simulink library "tramontina_database_moboticlib"  (R2024a)
settings: Solver=VariableStepAuto  StartTime=0.0  StopTime=10.0  RelTol=1e-3
libraries: canmsglib x4, simulink x1
settings Model: Creator=matlab.cut  LastModifiedBy=matlab.cut

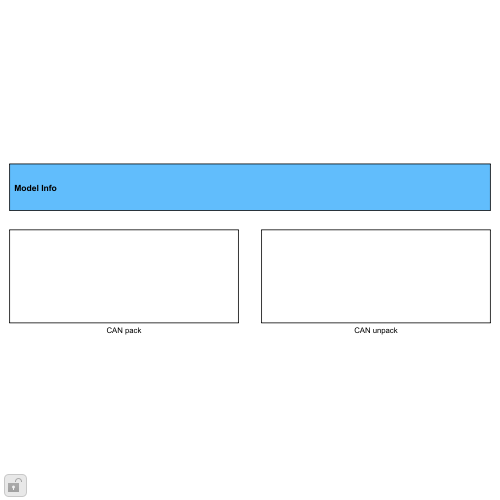
[thumbnail: Simulink's stored preview of the top-level diagram]
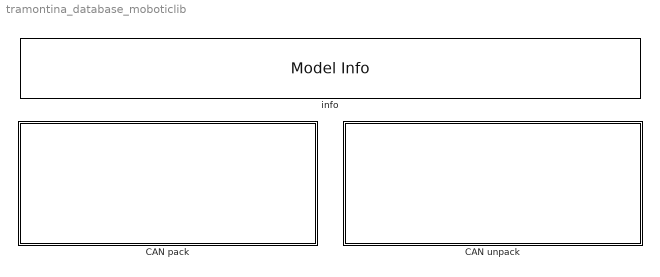
== system tramontina_database_moboticlib ==
  CAN pack : Subsystem
  CAN unpack : Subsystem
  info : simulink/Model-Wide Utilities/Model Info  Frame=on  DisplayStringWithTags=SPEEDGOAT CAN Database Library for: tramontina_database_mobotic  HorizontalTextAlignment=Left  LeftAlignmentValue=0.01

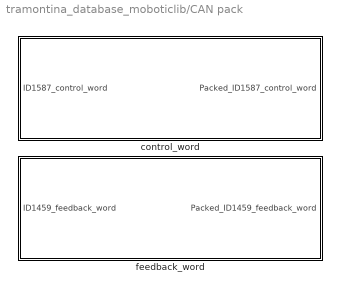
== system tramontina_database_moboticlib/CAN pack ==
  control_word : Subsystem
  feedback_word : Subsystem

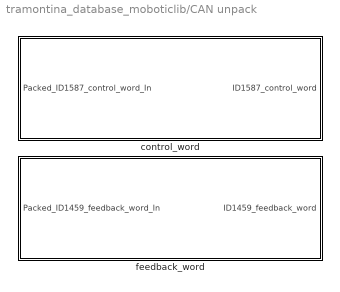
== system tramontina_database_moboticlib/CAN unpack ==
  control_word : Subsystem
  feedback_word : Subsystem

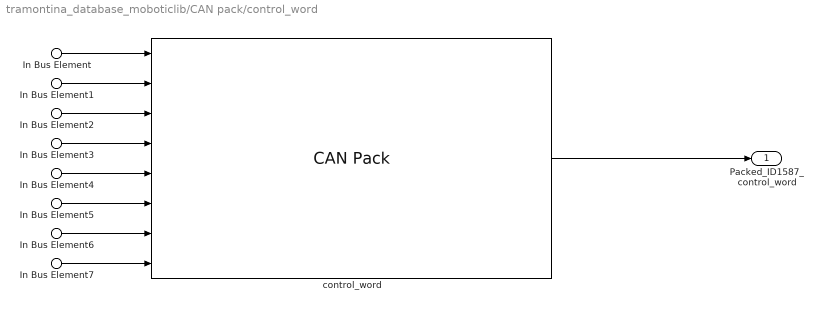
== system tramontina_database_moboticlib/CAN pack/control_word ==
  In Bus Element : Inport  PortName=ID1587_control_word  Element=byte0
  In Bus Element1 : Inport  PortName=ID1587_control_word  Element=byte1
  In Bus Element2 : Inport  PortName=ID1587_control_word  Element=byte2
  In Bus Element3 : Inport  PortName=ID1587_control_word  Element=byte3
  In Bus Element4 : Inport  PortName=ID1587_control_word  Element=byte4
  In Bus Element5 : Inport  PortName=ID1587_control_word  Element=byte5
  In Bus Element6 : Inport  PortName=ID1587_control_word  Element=byte6
  In Bus Element7 : Inport  PortName=ID1587_control_word  Element=byte7
  control_word : canmsglib/CAN Pack  CANdbFile=C:\Users\matlab.cut\Desktop\matlab\AMR_tramontina\Data\DBCFiles\tramontina_database_mobotic.dbc  MsgList=control_word  MsgName=control_word  MsgIDType=Standard (11-bit identifier)  MsgIdentifier=1587  MsgLength=8  Remote=off  ApplyMinMax=off  BusOutput=on  SignalInfo={'byte0','0','8','LE','unsigned','Standard','0','1','0','-Inf','Inf';'byte1','8','8','LE','unsigned','Standard','0','1','0','-Inf','Inf';'byte2','16','8','LE','unsigned','Standard','0','1','0','-Inf','Inf';'byte3','24','8','LE','unsigned','Standard','0','1','0','-Inf','Inf';'byte4','32','8','LE','unsigned','Standard','0','1','0','-Inf','Inf';'byte5','40','8','LE','unsigned','Standard','0','1','0','-Inf','Inf';'byte6','48','8','LE','unsigned','Standard','0','1','0','-Inf','Inf';'byte7','56','8','LE','unsigned','Standard','0','1','0','-Inf','Inf'}
      settings: DataFormat=manually specified signals
  Packed_ID1587_control_word : Outport
  wires:
  control_word/1 -> Packed_ID1587_control_word/1
  In Bus Element/1 -> control_word/1
  In Bus Element1/1 -> control_word/2
  In Bus Element2/1 -> control_word/3
  In Bus Element3/1 -> control_word/4
  In Bus Element4/1 -> control_word/5
  In Bus Element5/1 -> control_word/6
  In Bus Element6/1 -> control_word/7
  In Bus Element7/1 -> control_word/8

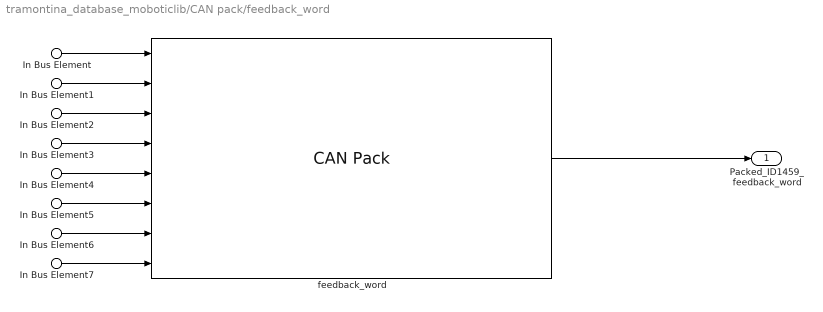
== system tramontina_database_moboticlib/CAN pack/feedback_word ==
  In Bus Element : Inport  PortName=ID1459_feedback_word  Element=byte0
  In Bus Element1 : Inport  PortName=ID1459_feedback_word  Element=byte1
  In Bus Element2 : Inport  PortName=ID1459_feedback_word  Element=byte2
  In Bus Element3 : Inport  PortName=ID1459_feedback_word  Element=byte3
  In Bus Element4 : Inport  PortName=ID1459_feedback_word  Element=byte4
  In Bus Element5 : Inport  PortName=ID1459_feedback_word  Element=byte5
  In Bus Element6 : Inport  PortName=ID1459_feedback_word  Element=byte6
  In Bus Element7 : Inport  PortName=ID1459_feedback_word  Element=byte7
  feedback_word : canmsglib/CAN Pack  CANdbFile=C:\Users\matlab.cut\Desktop\matlab\AMR_tramontina\Data\DBCFiles\tramontina_database_mobotic.dbc  MsgList=feedback_word  MsgName=feedback_word  MsgIDType=Standard (11-bit identifier)  MsgIdentifier=1459  MsgLength=8  Remote=off  ApplyMinMax=off  BusOutput=on  SignalInfo={'byte0','0','8','LE','unsigned','Standard','0','1','0','-Inf','Inf';'byte1','8','8','LE','unsigned','Standard','0','1','0','-Inf','Inf';'byte2','16','8','LE','unsigned','Standard','0','1','0','-Inf','Inf';'byte3','24','8','LE','unsigned','Standard','0','1','0','-Inf','Inf';'byte4','32','8','LE','unsigned','Standard','0','1','0','-Inf','Inf';'byte5','40','8','LE','unsigned','Standard','0','1','0','-Inf','Inf';'byte6','48','8','LE','unsigned','Standard','0','1','0','-Inf','Inf';'byte7','56','8','LE','unsigned','Standard','0','1','0','-Inf','Inf'}
      settings: DataFormat=manually specified signals
  Packed_ID1459_feedback_word : Outport
  wires:
  feedback_word/1 -> Packed_ID1459_feedback_word/1
  In Bus Element/1 -> feedback_word/1
  In Bus Element1/1 -> feedback_word/2
  In Bus Element2/1 -> feedback_word/3
  In Bus Element3/1 -> feedback_word/4
  In Bus Element4/1 -> feedback_word/5
  In Bus Element5/1 -> feedback_word/6
  In Bus Element6/1 -> feedback_word/7
  In Bus Element7/1 -> feedback_word/8

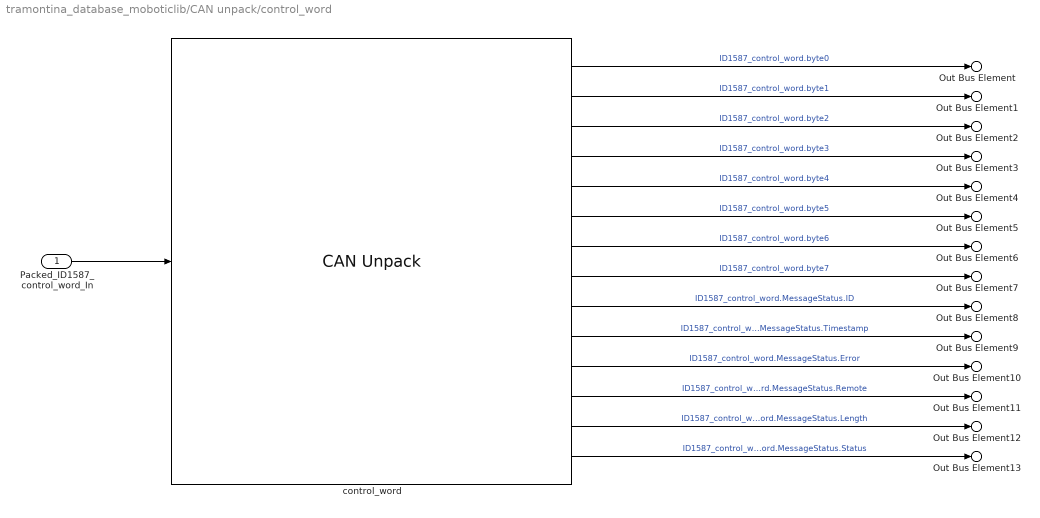
== system tramontina_database_moboticlib/CAN unpack/control_word ==
  Packed_ID1587_control_word_In : Inport
  control_word : canmsglib/CAN Unpack  CANdbFile=C:\Users\matlab.cut\Desktop\matlab\AMR_tramontina\Data\DBCFiles\tramontina_database_mobotic.dbc  MsgList=control_word  MsgName=control_word  MsgIDType=Standard (11-bit identifier)  MsgIdentifier=1587  MsgLength=8  SignalInfo={'byte0','0','8','LE','unsigned','Standard','0','1','0','-Inf','Inf';'byte1','8','8','LE','unsigned','Standard','0','1','0','-Inf','Inf';'byte2','16','8','LE','unsigned','Standard','0','1','0','-Inf','Inf';'byte3','24','8','LE','unsigned','Standard','0','1','0','-Inf','Inf';'byte4','32','8','LE','unsigned','Standard','0','1','0','-Inf','Inf';'byte5','40','8','LE','unsigned','Standard','0','1','0','-Inf','Inf';'byte6','48','8','LE','unsigned','Standard','0','1','0','-Inf','Inf';'byte7','56','8','LE','unsigned','Standard','0','1','0','-Inf','Inf'}  IDPort=on  TimestampPort=on  ErrorPort=on  RemotePort=on  LengthPort=on  StatusPort=on  ApplyMinMax=off
  Out Bus Element : Outport  PortName=ID1587_control_word  Element=byte0
  Out Bus Element1 : Outport  PortName=ID1587_control_word  Element=byte1
  Out Bus Element2 : Outport  PortName=ID1587_control_word  Element=byte2
  Out Bus Element3 : Outport  PortName=ID1587_control_word  Element=byte3
  Out Bus Element4 : Outport  PortName=ID1587_control_word  Element=byte4
  Out Bus Element5 : Outport  PortName=ID1587_control_word  Element=byte5
  Out Bus Element6 : Outport  PortName=ID1587_control_word  Element=byte6
  Out Bus Element7 : Outport  PortName=ID1587_control_word  Element=byte7
  Out Bus Element8 : Outport  PortName=ID1587_control_word  Element=MessageStatus.ID
  Out Bus Element9 : Outport  PortName=ID1587_control_word  Element=MessageStatus.Timestamp
  Out Bus Element10 : Outport  PortName=ID1587_control_word  Element=MessageStatus.Error
  Out Bus Element11 : Outport  PortName=ID1587_control_word  Element=MessageStatus.Remote
  Out Bus Element12 : Outport  PortName=ID1587_control_word  Element=MessageStatus.Length
  Out Bus Element13 : Outport  PortName=ID1587_control_word  Element=MessageStatus.Status
  wires:
  Packed_ID1587_control_word_In/1 -> control_word/1
  control_word/1 -> Out Bus Element/1  "ID1587_control_word.byte0"
  control_word/2 -> Out Bus Element1/1  "ID1587_control_word.byte1"
  control_word/3 -> Out Bus Element2/1  "ID1587_control_word.byte2"
  control_word/4 -> Out Bus Element3/1  "ID1587_control_word.byte3"
  control_word/5 -> Out Bus Element4/1  "ID1587_control_word.byte4"
  control_word/6 -> Out Bus Element5/1  "ID1587_control_word.byte5"
  control_word/7 -> Out Bus Element6/1  "ID1587_control_word.byte6"
  control_word/8 -> Out Bus Element7/1  "ID1587_control_word.byte7"
  control_word/9 -> Out Bus Element8/1  "ID1587_control_word.MessageStatus.ID"
  control_word/10 -> Out Bus Element9/1  "ID1587_control_word.MessageStatus.Timestamp"
  control_word/11 -> Out Bus Element10/1  "ID1587_control_word.MessageStatus.Error"
  control_word/12 -> Out Bus Element11/1  "ID1587_control_word.MessageStatus.Remote"
  control_word/13 -> Out Bus Element12/1  "ID1587_control_word.MessageStatus.Length"
  control_word/14 -> Out Bus Element13/1  "ID1587_control_word.MessageStatus.Status"

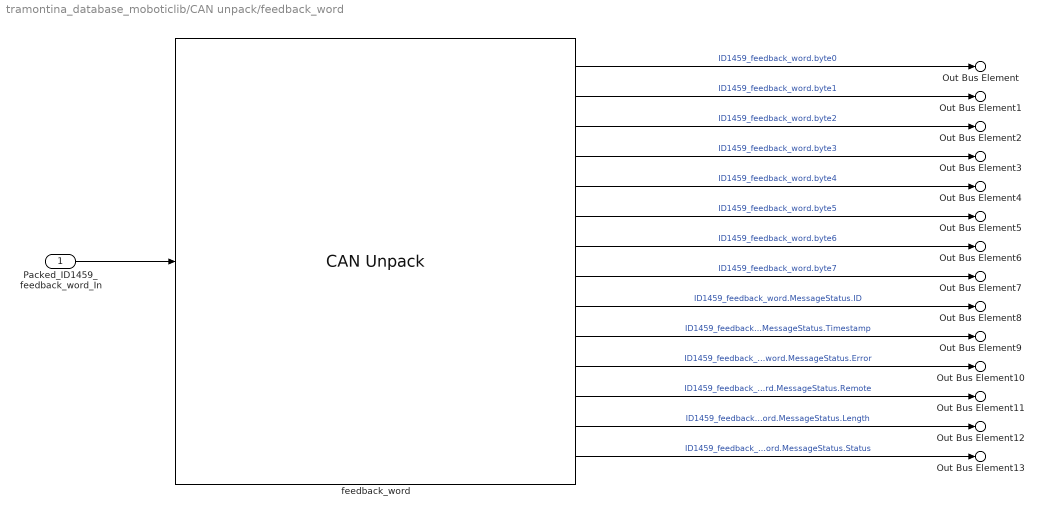
== system tramontina_database_moboticlib/CAN unpack/feedback_word ==
  Packed_ID1459_feedback_word_In : Inport
  feedback_word : canmsglib/CAN Unpack  CANdbFile=C:\Users\matlab.cut\Desktop\matlab\AMR_tramontina\Data\DBCFiles\tramontina_database_mobotic.dbc  MsgList=feedback_word  MsgName=feedback_word  MsgIDType=Standard (11-bit identifier)  MsgIdentifier=1459  MsgLength=8  SignalInfo={'byte0','0','8','LE','unsigned','Standard','0','1','0','-Inf','Inf';'byte1','8','8','LE','unsigned','Standard','0','1','0','-Inf','Inf';'byte2','16','8','LE','unsigned','Standard','0','1','0','-Inf','Inf';'byte3','24','8','LE','unsigned','Standard','0','1','0','-Inf','Inf';'byte4','32','8','LE','unsigned','Standard','0','1','0','-Inf','Inf';'byte5','40','8','LE','unsigned','Standard','0','1','0','-Inf','Inf';'byte6','48','8','LE','unsigned','Standard','0','1','0','-Inf','Inf';'byte7','56','8','LE','unsigned','Standard','0','1','0','-Inf','Inf'}  IDPort=on  TimestampPort=on  ErrorPort=on  RemotePort=on  LengthPort=on  StatusPort=on  ApplyMinMax=off
  Out Bus Element : Outport  PortName=ID1459_feedback_word  Element=byte0
  Out Bus Element1 : Outport  PortName=ID1459_feedback_word  Element=byte1
  Out Bus Element2 : Outport  PortName=ID1459_feedback_word  Element=byte2
  Out Bus Element3 : Outport  PortName=ID1459_feedback_word  Element=byte3
  Out Bus Element4 : Outport  PortName=ID1459_feedback_word  Element=byte4
  Out Bus Element5 : Outport  PortName=ID1459_feedback_word  Element=byte5
  Out Bus Element6 : Outport  PortName=ID1459_feedback_word  Element=byte6
  Out Bus Element7 : Outport  PortName=ID1459_feedback_word  Element=byte7
  Out Bus Element8 : Outport  PortName=ID1459_feedback_word  Element=MessageStatus.ID
  Out Bus Element9 : Outport  PortName=ID1459_feedback_word  Element=MessageStatus.Timestamp
  Out Bus Element10 : Outport  PortName=ID1459_feedback_word  Element=MessageStatus.Error
  Out Bus Element11 : Outport  PortName=ID1459_feedback_word  Element=MessageStatus.Remote
  Out Bus Element12 : Outport  PortName=ID1459_feedback_word  Element=MessageStatus.Length
  Out Bus Element13 : Outport  PortName=ID1459_feedback_word  Element=MessageStatus.Status
  wires:
  Packed_ID1459_feedback_word_In/1 -> feedback_word/1
  feedback_word/1 -> Out Bus Element/1  "ID1459_feedback_word.byte0"
  feedback_word/2 -> Out Bus Element1/1  "ID1459_feedback_word.byte1"
  feedback_word/3 -> Out Bus Element2/1  "ID1459_feedback_word.byte2"
  feedback_word/4 -> Out Bus Element3/1  "ID1459_feedback_word.byte3"
  feedback_word/5 -> Out Bus Element4/1  "ID1459_feedback_word.byte4"
  feedback_word/6 -> Out Bus Element5/1  "ID1459_feedback_word.byte5"
  feedback_word/7 -> Out Bus Element6/1  "ID1459_feedback_word.byte6"
  feedback_word/8 -> Out Bus Element7/1  "ID1459_feedback_word.byte7"
  feedback_word/9 -> Out Bus Element8/1  "ID1459_feedback_word.MessageStatus.ID"
  feedback_word/10 -> Out Bus Element9/1  "ID1459_feedback_word.MessageStatus.Timestamp"
  feedback_word/11 -> Out Bus Element10/1  "ID1459_feedback_word.MessageStatus.Error"
  feedback_word/12 -> Out Bus Element11/1  "ID1459_feedback_word.MessageStatus.Remote"
  feedback_word/13 -> Out Bus Element12/1  "ID1459_feedback_word.MessageStatus.Length"
  feedback_word/14 -> Out Bus Element13/1  "ID1459_feedback_word.MessageStatus.Status"
